simulink model "Open_vs_Closed_Loop"  (R2023b)
settings: Solver=VariableStepAuto  StartTime=0.0  StopTime=10.0  RelTol=1e-3
undefined symbols (not defined in the file): Wn, zeta
settings Model: Creator=ascom  LastModifiedBy=ascom

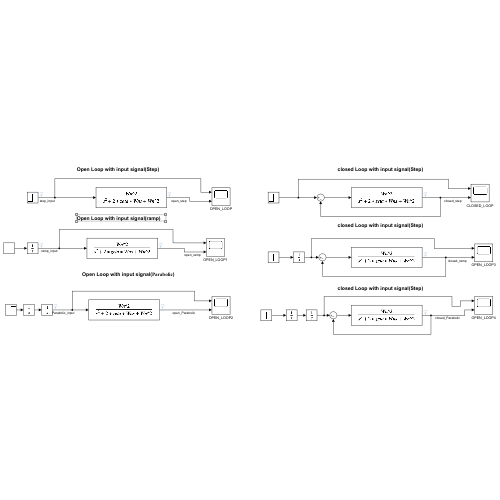
[thumbnail: Simulink's stored preview of the top-level diagram]
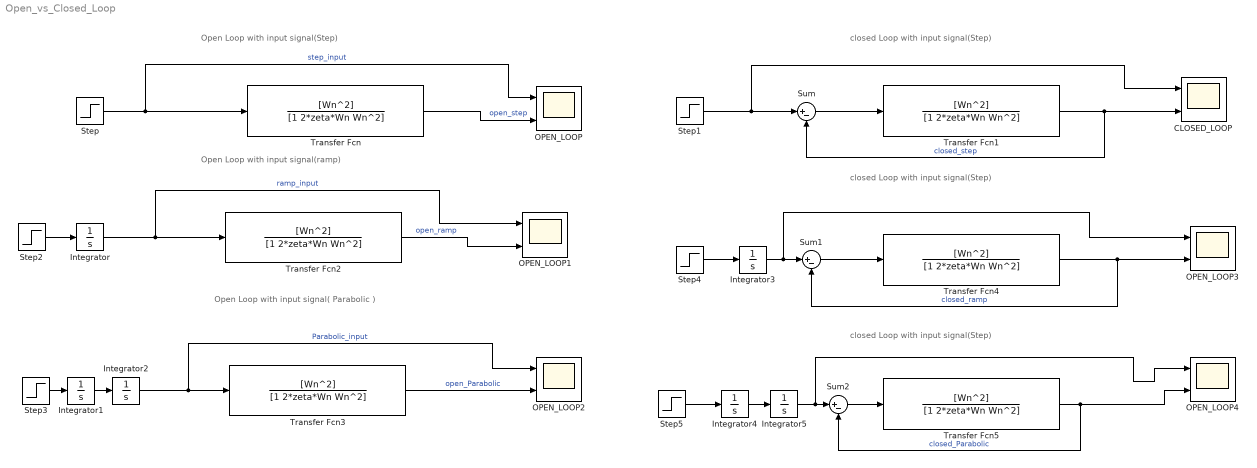
== system Open_vs_Closed_Loop ==
  note: Open Loop with input signal(Step)
  note: Open Loop with input signal(ramp)
  note: Open Loop with input signal( Parabolic )
  note: closed Loop with input signal(Step)
  note: closed Loop with input signal(Step)
  note: closed Loop with input signal(Step)
  CLOSED_LOOP : Scope  NumInputPorts=2
  Integrator{,1..5} (6 alike) : Integrator
  OPEN_LOOP{,1..4} (5 alike) : Scope  NumInputPorts=2
  Step{,1..5} (6 alike) : Step  SampleTime=0
  Sum : Sum  Inputs=|+-
  Sum1 : Sum  Inputs=|+-
  Sum2 : Sum  Inputs=|+-
  Transfer Fcn{,1..5} (6 alike) : TransferFcn  Numerator=[Wn^2]  Denominator=[1 2*zeta*Wn Wn^2]
  wires:
  Transfer Fcn/1 -> OPEN_LOOP/2  "open_step"
  Step/1 -> OPEN_LOOP/1, Transfer Fcn/1  "step_input"
  Step1/1 -> CLOSED_LOOP/1, Sum/1
  Sum/1 -> Transfer Fcn1/1
  Transfer Fcn1/1 -> CLOSED_LOOP/2, Sum/2  "closed_step"
  Step2/1 -> Integrator/1
  Transfer Fcn2/1 -> OPEN_LOOP1/2  "open_ramp"
  Integrator/1 -> OPEN_LOOP1/1, Transfer Fcn2/1  "ramp_input"
  Transfer Fcn3/1 -> OPEN_LOOP2/2  "open_Parabolic"
  Step3/1 -> Integrator1/1
  Integrator1/1 -> Integrator2/1
  Integrator2/1 -> OPEN_LOOP2/1, Transfer Fcn3/1  "Parabolic_input"
  Transfer Fcn4/1 -> Sum1/2, OPEN_LOOP3/2  "closed_ramp"
  Step4/1 -> Integrator3/1
  Integrator4/1 -> Integrator5/1
  Step5/1 -> Integrator4/1
  Transfer Fcn5/1 -> OPEN_LOOP4/2, Sum2/2  "closed_Parabolic"
  Integrator3/1 -> OPEN_LOOP3/1, Sum1/1
  Sum1/1 -> Transfer Fcn4/1
  Integrator5/1 -> OPEN_LOOP4/1, Sum2/1
  Sum2/1 -> Transfer Fcn5/1
